simulink model "ThreePhaseVectorControl v2"  (R2020a)
settings: Solver=ode15s  StartTime=0.0  StopTime=2.5  MaxStep=1e-6  RelTol=1e-6
model workspace (MAT data in the model file):
  frequency = 1
values from neighbouring files (symbols this model uses):
  Buffer = 500    [PLLFYP.m]
  Ki_PLL = 0.005    [PLLFYP.m]
  Kp_PLL = 0.05    [PLLFYP.m]
  Kp_VSC = 500    [PLLFYP.m]
  Lf = 0.005    [PLLFYP.m]
  Lg = XR*Rg/(100*pi)    [PLLFYP.m]
  MPM_Ts = 1/5000    (= 0.0002)    [PLLFYP.m]
  Rf = 0.1    [PLLFYP.m]
  Rg = sqrt((1/(1+XR^2))*((500^2)/(Pn*SCR))^2)    [PLLFYP.m]
  Vdc = 2000    [PLLFYP.m]
  wL = 2*pi*50*Lf    (= 1.57079632679)    [PLLFYP.m]
  wn = 3000    [PLLFYP.m]
  zeta = 0.707    [PLLFYP.m]
undefined symbols (not defined in the file or in its folder): Ki_PQ, Kp_PQ, mpm_wc, plecs, Q, Q_KF, R, wb, wc, wc1, wc2
libraries: powerlib_meascontrol x57, powerlib x25, simulink x4, eeStairGenerator x4, powerlib_extras x2, cstblocks x2
(part 4 of 4)

== matlab function ThreePhaseVectorControl v2/Vector Current Controller + PWM/CF/MATLAB Function1 ==
  settings: updateMethod=DISCRETE
  data: G1 output; ROCOF input; clk input; G2 output
function [G1, G2]  = fcn(ROCOF, clk)

persistent time; persistent trig; persistent prev_G;   

if isempty(time)        % Initialize variables
    time = 0;
end
if isempty(trig)
    trig = 0;
end
if isempty(prev_G)
    prev_G = 0;
end

threshold = 2300;       % Set threshold to categorize dynamic/steady state

if (ROCOF < threshold)  % Steady state
    G1 = 0;
else 
    G1 = 1;             % dynamic
end

if (prev_G > G1)&&(trig == 0)       % Condition for switching from dynamic to steady state
    time = clk;
    G1 = 1;
    trig = 1;
elseif (prev_G > G1)&&(clk < time + 0.1)&&(trig == 1)   % Wait 0.1s before switching
    G1 = 1;
elseif (prev_G > G1)&&(clk == time + 0.1)&&(trig == 1)  % Switch
    G1 = 0;
    trig = 0;
elseif (prev_G == G1)&&(trig == 1)      % Start clock again if another dynamic event occurs
    time = clk;
end

G2 = 1 - G1;
prev_G = G1;

end

== matlab function ThreePhaseVectorControl v2/Vector Current Controller + PWM/CF/MATLAB Function2 ==
  data: G1 output; ROCOF input; G2 output
function [G1, G2] = fcn(ROCOF)

min_threshold = 1800;
max_threshold = 3500;

if (ROCOF < min_threshold)  % Steady state
    G1 = 0;
elseif (min_threshold <= ROCOF)&&(ROCOF < max_threshold)
    G1 = (ROCOF - min_threshold)/(max_threshold - min_threshold);
else 
    G1 = 1;
end

G2 = 1 - G1; % MPM weight

end

== matlab function ThreePhaseVectorControl v2/Vector Current Controller + PWM/KF_PLL/Kalman Filter-based PLL/Kalman Filter/KF_Vb ==
  data: Vb input; Vbk_S90 output; R input; Q input; w_k input; w_fk input
function Vbk_S90   = fcn(Vb, R, Q, w_k, w_fk)
 
persistent Phat;
persistent xhat;
 
if isempty(Phat)
      Phat = eye(6);
end
if isempty(xhat)
      xhat = zeros(6);
end

 
Ts = 10e-6;
 
a = sin(w_k*Ts)*sin(w_fk*Ts);
b = cos(w_k*Ts)*cos(w_fk*Ts);
c = sin(w_k*Ts)*cos(w_fk*Ts);
d = cos(w_k*Ts)*sin(w_fk*Ts);
e = sin(w_k*Ts);
f = cos(w_k*Ts);
phi_k = [b a d c 0 0; -a b -c -d 0 0; -d c b -a 0 0; -c d a b 0 0; 0 0 0 0 f e; 0 0 0 0 -e f];
F_k = [1 0 0 0 1 0];
 
% Time update
xhat_next = phi_k * xhat;
Phat_next = phi_k * Phat * phi_k' + Q;

% Kalman gain
K_k = 0.005*Phat_next * F_k' * inv(F_k*Phat_next*F_k' + R);

% Measurement update
xhat = xhat_next + K_k*(Vb - F_k*xhat_next);
Phat = Phat_next - K_k*F_k*Phat_next;

Vbk_S90 = xhat(6);

%K_k = phi_k * Phat * F_k' * (F_k*Phat*F_k' + R)^(-1);       % Compute Kalman gain
%xhat_next = phi_k * xhat + K_k*(Vb - F_k * xhat);           % Next state
%Phat_next = phi_k*Phat*phi_k' - K_k*F_k*Phat*phi_k' + ones(6)*Q;    % Predict state covariance
 
%Vbk_S90 = xhat_next(6);
 
%Phat = Phat_next;
%xhat = xhat_next;
 
end

== matlab function ThreePhaseVectorControl v2/Vector Current Controller + PWM/KF_PLL/Kalman Filter-based PLL/Kalman Filter/KF_Vc ==
  data: Vck_S90 output; Vc input; R input; Q input; w_k input; w_fk input
function Vck_S90  = fcn(Vc, R, Q, w_k, w_fk)
 
persistent Phat;
persistent xhat;
 
if isempty(Phat)
        Phat = eye(6);
end
if isempty(xhat)
        xhat = zeros(6);
end

Ts = 10e-6;
 
a = sin(w_k*Ts)*sin(w_fk*Ts);
b = cos(w_k*Ts)*cos(w_fk*Ts);
c = sin(w_k*Ts)*cos(w_fk*Ts);
d = cos(w_k*Ts)*sin(w_fk*Ts);
e = sin(w_k*Ts);
f = cos(w_k*Ts);
phi_k = [b a d c 0 0; -a b -c -d 0 0; -d c b -a 0 0; -c d a b 0 0; 0 0 0 0 f e; 0 0 0 0 -e f];
F_k = [1 0 0 0 1 0];

% Time update
xhat_next = phi_k * xhat;
Phat_next = phi_k * Phat * phi_k' + Q;

% Kalman gain
K_k = 0.005*Phat_next * F_k' * inv(F_k*Phat_next*F_k' + R);

% Measurement update
xhat = xhat_next + K_k*(Vc - F_k*xhat_next);
Phat = Phat_next - K_k*F_k*Phat_next;

Vck_S90 = xhat(6);

%K_k = phi_k * Phat * F_k' * (F_k*Phat*F_k' + R)^(-1);       % Compute Kalman gain
%xhat_next = phi_k * xhat + K_k*(Vc - F_k * xhat);           % Next state
%Phat_next = phi_k*Phat*phi_k' - K_k*F_k*Phat*phi_k' + ones(6)*Q;    % Predict state covariance
 
%Vck_S90 = xhat_next(6);
 
%x1k = xhat_next(1);                 % Flicker disturbance at n=1 freq
%x2k = xhat_next(2);                 % Flicker disturbance at n=2 freq
%x3k = xhat_next(3);                 % Flicker disturbance at n=3 freq
%x4k = xhat_next(4);                 % Flicker disturbance at n=4 freq
 
%Phat = Phat_next;
%xhat = xhat_next;
 
end

== matlab function ThreePhaseVectorControl v2/Vector Current Controller + PWM/FFT_PLL/FFT PLL ==
  data: data input; f output; T input
function f = fcn(data, T)

%data = detrend(data,0);

f = 0;

Fs = 1/T;
N = length(data);

NFFT = 2^nextpow2(N); % Next power of 2 from length of y
Y = fft(data,NFFT)/N;
fz = Fs/2*linspace(0,1,NFFT/2+1);
Y_new = 2*abs(Y(1:NFFT/2+1));

[temp, i] = max(Y_new);
f = fz(i);





% NFFT = 2 ^ nextpow2(N);             % Compute FFT length
% Y = fft(data, NFFT);   % Compute FFT of signal
% Y = Y(1:NFFT/2);                    % Take one side of FFT plot
% Y_abs = 1/NFFT*abs(Y);              % Calculate magnitude and normalize the spectrum
% f_fft = (0:NFFT/2-1)*Fs/NFFT;       % Scale the frequency axis
% 
% [m, i] = max(Y_abs);    % Find peak frequency
% % % 
% f = f_fft(i);           % Output the corresponding frequency of the peak


% f = 0;
% 
% T = 10e-6;
% Fs = 1/T;
% L = size(data,1);
% 
% Y = fft(data);
% Y = abs(Y/L);
% X = Y(1:L/2+1);
% X(2:end-1) = 2*X(2:end-1);
% fr = Fs*(0:(L/2))/L;
% 
% %plot(fr, X)          % Plot frequency
% 
% [m, i] = max(X);     % Find peak frequency
% 
% f = fr(i);           % Output the corresponding frequency of the peak

== matlab function ThreePhaseVectorControl v2/Vector Current Controller + PWM/KF_PLL/KF//GAM/Kalman Filter/KF_Va ==
  data: y_k input; v_fk output; R input; Q input; w_k input; V_fk_S90 output
function [v_fk, V_fk_S90] = fcn(y_k, R, Q, w_k)
 
persistent P_k;
persistent xhat_k;

% Initialize xhat and Phat
    if isempty(P_k)
        P_k = eye(2, 2); %eye(2);
    end
    if isempty(xhat_k)
        xhat_k = zeros(2, 1);
    end
    
% Variables for KF
    Ts = 10e-6;       
    phi_k = [cos(w_k*Ts) sin(w_k*Ts); -sin(w_k*Ts) cos(w_k*Ts)]; 
    F_k = [1 0];


K = phi_k * P_k * F_k' / (F_k * P_k * F_k' + R);        %K_gain * Phat_next * F_k' /(F_k*Phat_next*F_k' + R);    
xhat_k1 = phi_k * xhat_k + K * (y_k - F_k * xhat_k);
P_k1 = phi_k * P_k * phi_k' - K * F_k * P_k * phi_k' + Q;

xhat_k = xhat_k1;
P_k = P_k1;

% Output
v_fk = xhat_k1(1);
V_fk_S90 = xhat_k1(2);


 
end

== matlab function ThreePhaseVectorControl v2/Vector Current Controller + PWM/KF_PLL/Kalman Filter-based PLL/Kalman Filter/KF_Va ==
  data: Va input; Vak_S90 output; R input; Q input; w_k input; w_fk input
function Vak_S90    = fcn(Va, R, Q, w_k, w_fk)
 
persistent Phat;
persistent xhat;

if isempty(Phat)
    Phat = eye(6);
end
if isempty(xhat)
    xhat = zeros(6);
end


Ts = 10e-6;
 
a = sin(w_k*Ts)*sin(w_fk*Ts);
b = cos(w_k*Ts)*cos(w_fk*Ts);
c = sin(w_k*Ts)*cos(w_fk*Ts);
d = cos(w_k*Ts)*sin(w_fk*Ts);
e = sin(w_k*Ts);
f = cos(w_k*Ts);
phi_k = [b a d c 0 0; -a b -c -d 0 0; -d c b -a 0 0; -c d a b 0 0; 0 0 0 0 f e; 0 0 0 0 -e f];
F_k = [1 0 0 0 1 0];
 
% Time update
xhat_next = phi_k * xhat;
Phat_next = phi_k * Phat * phi_k' + Q;

% Kalman gain
K_k = 0.005*Phat_next * F_k' * inv(F_k*Phat_next*F_k' + R);

% Measurement update
xhat = xhat_next + K_k*(Va - F_k*xhat_next);
Phat = Phat_next - K_k*F_k*Phat_next;

Vak_S90 = xhat(6);



%K_k = phi_k * Phat * F_k' * (F_k*Phat*F_k' + R)^(-1);       % Compute Kalman gain
%xhat_next = phi_k * xhat + K_k*(Va - F_k * xhat);           % Next state
%Phat_next = phi_k*Phat*phi_k' - K_k*F_k*Phat*phi_k' + ones(6)*Q;    % Predict state covariance

%Vak_S90 = xhat_next(6);

%Phat = Phat_next;
%xhat = xhat_next;
 
end

== matlab function ThreePhaseVectorControl v2/Vector Current Controller + PWM/CF based on i_d/CF_func ==
  data: i_d input; MPM input; SRF input; CF_freq output; FFT_freq input
function CF_freq = fcn(i_d, MPM, SRF, FFT_freq)

g1 = 0;
g2 = 0;

if (i_d < 10)
    g1 = 1;
    g2 = 0;
elseif (10 <= i_d)&&(i_d < 15)
    g1 = 0;
    g2 = 0;
elseif (15 <= i_d)&&(i_d < 20)
    g1 = 0;
    g2 = (i_d-15)/5;
else
    g1 = 0;
    g2 = 1;
end

f = g1 * SRF + (1-g1-g2) * MPM + g2 * FFT_freq;

CF_freq = f;

== matlab function ThreePhaseVectorControl v2/Vector Current Controller + PWM/MPM CF/MPM/MPM 0.5 cycle ==
  data: x input; L input; timestep input; freq_guess input; outputfreq output; cycle5_freq input
function outputfreq = Our_MPM_QR_pca(x,L,timestep,freq_guess, cycle5_freq)

%     Applies the Total Forward Backward Matrix Pencil Method to resolve the
%     synchrophasor of an input signal
%     Author: Lakshan Bernard, Sunny Goondram

% Inputs
% x:          one window of the timeseries
% L:          pencil parameter
% timestep:   time between sample points
% freq_guess: which phasors to report. NB: the method calculates all phasors
%             but the this just tells the algorithm to output phasor closest
%             to freq_guess
%             
% Outputs
% outputphasor:   a complex number representing the phasor relative to start
%                 of the window.
% outputfreq:     the frequency of the phasor. Note this is different to
%                 freq_guess
% eigS, residues: these contain all the frequency and phasor data

x = reshape(x, [], 1); %reshape data into column vector
N = length(x);
sampleoffset = (ceil(N/2)+1);
xold = x;

persistent f0;
if isempty(f0)
    f0 = freq_guess;
end

% Hyperparameters
DYNAMIC = 0;
if(DYNAMIC)
    epsilon=0.125;
    sys_order=floor((0.22/(50*timestep)));
else
    epsilon= 0.725;  %0.0050;
    sys_order=floor((N-sampleoffset)*1);
end

%% Filtering
    L1 = ceil(N/2);
    Y = hankel(x(1:N-L1), x(N-L1:N)); diagIdx = (N:-1:1)-L1;
    
    Y_mean = mean(Y,1);
    n = size(Y,1);
    matrix_mean = repmat(Y_mean,n,1); %creates a matrix with similar rows 
    centered_data = Y- matrix_mean;% centering the data by subtracting the mean
    M = ((centered_data')*centered_data)/(n-1);
    [V,D] = eig(M); %V are eigenvectors and D represents the eigenvalues 

    %sorting the eigen values in descending order
    lx = size(Y,2);
    eval = zeros(1,lx);
    eval = complex(eval, zeros(size(eval), class(eval)) );                      % Additional code added in
    for k = 1:lx
        eval(1,k) = D(k,k);
    end 
    [eval_sorted,I] = sort(eval,'descend');
    
    S = cumsum(abs(eval_sorted));
    limit = find((S/S(end))>0.9999999,1);
    if isempty(limit)                                                           % Additional code added in
        limit = 1;
    end
    limit = limit(1);
    evec_sorted = zeros(lx,limit);
    evec_sorted = complex(evec_sorted, zeros(size(evec_sorted), class(evec_sorted)) );    % Additional code added in
    for m =1:limit
        evec_sorted(:,m) = V(:,I(m));
    end
        
    %reconstruction
    princ_compon_limit = centered_data*evec_sorted;
    reconstructed = princ_compon_limit *(evec_sorted');
    reconstructed = reconstructed + matrix_mean;
    C = reconstructed;
 
    x1 = zeros(1,N);
    x1 = complex(x1, zeros(size(x1), class(x1)) );                              % Additional code added in
    for i=1:length(diagIdx) %averaging antidiagonals
        x1(i) = mean(diag(fliplr(C),diagIdx(i)));
    end    
    C = hankel(x1(1:N-L1), x1(N-L1:N)); 

    
%% Solving GEP

%perform the Column permutated QR decomposition for finding eigenvalues
%find the QR decomp for the all data matrix
[Q,R,E]=qr(C);

%rank estimation
order=0;

for i=1:length(diag(R))
    if abs(R(i,i))>=epsilon*abs(R(1,1))
        order=order+1;
    end
end

% Use permutation matrix to modify the Triangular R matrix
S=R*((E).');
% Create a new truncated pencil using the new matrix 
T1=S(1:order,1:L);
T2=S(1:order,2:L+1);
%modify the new pencil with diagonal of R matrix
Dinv=inv(diag(diag(R(1:order,1:order))));
T1dash=Dinv*T1;
T2dash=Dinv*T2;
%use the new pencil to find the eigenvalues
eigsS=eig(pinv(T2dash)*T1dash);
%remove the 0 eigenvalues;

eigsS(abs(eigsS)<10^-8)=[];
eigsS((abs(eigsS)<0.9)|(abs(eigsS)>1.1))=0;
order=length(eigsS);

%% Solving Complex Amplitudes
%form the linear system to solve for the complex amplitudes
ans_vec=xold(1+sampleoffset:sys_order+sampleoffset); %build answer vector (NB, this data hasnt been filtered :/)
coef_mat=zeros(sys_order,order);
coef_mat = complex(coef_mat, zeros(size(coef_mat), class(coef_mat)) );         % Additional code added in
for i=1:sys_order %build coefficient matrix
    for j=1:order
        coef_mat(i,j)=eigsS(j)^(i-1);
    end
end
residues=pinv(coef_mat)*ans_vec; %find the complex amplitudes


%% Estimating Frequency
freq = angle(eigsS)/(2*pi*timestep);
estfreq=freq_guess; %to report fundamental phasor replace with 50..
outputfreq_temp = mean(freq( (freq>0.2*estfreq)&(freq<2.0*estfreq) )); %mean(freq( (freq>0.85*estfreq)&(freq<1.15*estfreq) ));

if (outputfreq_temp < 100)&&(outputfreq_temp > 0)
    f0 = outputfreq_temp;
else
    outputfreq_temp = cycle5_freq;
end
 
 outputfreq = outputfreq_temp;

%% Reconstructing Phasor
%outputphasor = 2*sum(residues( (freq>0.85*freq_guess)&(freq<1.15*freq_guess) ));

== matlab function ThreePhaseVectorControl v2/Vector Current Controller + PWM/MPM CF/MPM/MPM 5 cycle ==
  data: x input; L input; timestep input; freq_guess input; outputfreq output
function outputfreq = Our_MPM_QR_pca(x,L,timestep,freq_guess)

%     Applies the Total Forward Backward Matrix Pencil Method to resolve the
%     synchrophasor of an input signal
%     Author: Lakshan Bernard, Sunny Goondram

% Inputs
% x:          one window of the timeseries
% L:          pencil parameter
% timestep:   time between sample points
% freq_guess: which phasors to report. NB: the method calculates all phasors
%             but the this just tells the algorithm to output phasor closest
%             to freq_guess
%             
% Outputs
% outputphasor:   a complex number representing the phasor relative to start
%                 of the window.
% outputfreq:     the frequency of the phasor. Note this is different to
%                 freq_guess
% eigS, residues: these contain all the frequency and phasor data

x = reshape(x, [], 1); %reshape data into column vector
N = length(x);
sampleoffset = (ceil(N/2)+1);
xold = x;

% Hyperparameters
DYNAMIC = 0;
if(DYNAMIC)
    epsilon=0.125;
    sys_order=floor((0.22/(50*timestep)));
else
    epsilon=0.725; %0.0050;
    sys_order=floor((N-sampleoffset)*1);
end

%% Filtering
    L1 = ceil(N/2);
    Y = hankel(x(1:N-L1), x(N-L1:N)); diagIdx = (N:-1:1)-L1;
    
    Y_mean = mean(Y,1);
    n = size(Y,1);
    matrix_mean = repmat(Y_mean,n,1); %creates a matrix with similar rows 
    centered_data = Y- matrix_mean;% centering the data by subtracting the mean
    M = ((centered_data')*centered_data)/(n-1);
    [V,D] = eig(M); %V are eigenvectors and D represents the eigenvalues 

    %sorting the eigen values in descending order
    lx = size(Y,2);
    eval = zeros(1,lx);
    eval = complex(eval, zeros(size(eval), class(eval)) );                      % Additional code added in
    for k = 1:lx
        eval(1,k) = D(k,k);
    end 
    [eval_sorted,I] = sort(eval,'descend');
    
    S = cumsum(abs(eval_sorted));
    limit = find((S/S(end))>0.9999999,1);
    if isempty(limit)                                                           % Additional code added in
        limit = 1;
    end
    limit = limit(1);
    evec_sorted = zeros(lx,limit);
    evec_sorted = complex(evec_sorted, zeros(size(evec_sorted), class(evec_sorted)) );    % Additional code added in
    for m =1:limit
        evec_sorted(:,m) = V(:,I(m));
    end
        
    %reconstruction
    princ_compon_limit = centered_data*evec_sorted;
    reconstructed = princ_compon_limit *(evec_sorted');
    reconstructed = reconstructed + matrix_mean;
    C = reconstructed;
 
    x1 = zeros(1,N);
    x1 = complex(x1, zeros(size(x1), class(x1)) );                              % Additional code added in
    for i=1:length(diagIdx) %averaging antidiagonals
        x1(i) = mean(diag(fliplr(C),diagIdx(i)));
    end    
    C = hankel(x1(1:N-L1), x1(N-L1:N)); 

    
%% Solving GEP

%perform the Column permutated QR decomposition for finding eigenvalues
%find the QR decomp for the all data matrix
[Q,R,E]=qr(C);

%rank estimation
order=0;

for i=1:length(diag(R))
    if abs(R(i,i))>=epsilon*abs(R(1,1))
        order=order+1;
    end
end

% Use permutation matrix to modify the Triangular R matrix
S=R*((E).');
% Create a new truncated pencil using the new matrix 
T1=S(1:order,1:L);
T2=S(1:order,2:L+1);
%modify the new pencil with diagonal of R matrix
Dinv=inv(diag(diag(R(1:order,1:order))));
T1dash=Dinv*T1;
T2dash=Dinv*T2;
%use the new pencil to find the eigenvalues
eigsS=eig(pinv(T2dash)*T1dash);
%remove the 0 eigenvalues;

eigsS(abs(eigsS)<10^-8)=[];
eigsS((abs(eigsS)<0.9)|(abs(eigsS)>1.1))=0;
order=length(eigsS);

%% Solving Complex Amplitudes
%form the linear system to solve for the complex amplitudes
ans_vec=xold(1+sampleoffset:sys_order+sampleoffset); %build answer vector (NB, this data hasnt been filtered :/)
coef_mat=zeros(sys_order,order);
coef_mat = complex(coef_mat, zeros(size(coef_mat), class(coef_mat)) );         % Additional code added in
for i=1:sys_order %build coefficient matrix
    for j=1:order
        coef_mat(i,j)=eigsS(j)^(i-1);
    end
end
residues=pinv(coef_mat)*ans_vec; %find the complex amplitudes


%% Estimating Frequency
freq = angle(eigsS)/(2*pi*timestep);
estfreq=freq_guess; %to report fundamental phasor replace with 50..
outputfreq = mean(freq( (freq>0.85*estfreq)&(freq<1.15*estfreq) ));

%% Reconstructing Phasor
%outputphasor = 2*sum(residues( (freq>0.85*freq_guess)&(freq<1.15*freq_guess) ));

== matlab function ThreePhaseVectorControl v2/Vector Current Controller + PWM/KF_PLL/KF//GAM/Kalman Filter/KF_Va1 ==
  data: Va input; Vb input; Vc input; Vak output; R input; Q input; w_k input; Vbk output; Vck output; K_gain input
function [Vak, Vbk, Vck] = fcn(Va, Vb, Vc, R, Q, w_k, K_gain)
 
persistent Phat_a; persistent Phat_b; persistent Phat_c;
persistent xhat_a; persistent xhat_b; persistent xhat_c;

% Initialize xhat and Phat
    if isempty(Phat_a)
        Phat_a = eye(2);
    end
    if isempty(Phat_b)
        Phat_b = eye(2);
    end
    if isempty(Phat_c)
        Phat_c = eye(2);
    end
    if isempty(xhat_a)
        xhat_a = zeros(2, 1);
    end
    if isempty(xhat_b)
        xhat_b = zeros(2, 1);
    end
    if isempty(xhat_c)
        xhat_c = zeros(2, 1);
    end
    
% Initialize w_k to 2*pi*50 for 40us
%     if isempty(w_k)
%         w_k = 2*pi*50;
%     end

% Variables & matrices for KF
    Ts = 10e-6;        % time period = 10 us
    phi_k = [cos(w_k*Ts) sin(w_k*Ts); -sin(w_k*Ts) cos(w_k*Ts)];  %phi_k = [1 0; 0 1];
    F_k = [1 0];

%%%%%%%%%%%%%%%%%%%%% KF for Va %%%%%%%%%%%%%%%%%%%%%
% Time update
xhat_a_next = phi_k * xhat_a;
Phat_a_next = phi_k * Phat_a * phi_k' + Q;

% Kalman gain
K_a = K_gain*Phat_a_next * F_k' /(F_k*Phat_a_next*F_k' + R);

% Measurement update
xhat_a = xhat_a_next + K_a*(Va - F_k*xhat_a_next);
Phat_a = Phat_a_next - K_a*F_k*Phat_a_next;


%%%%%%%%%%%%%%%%%%%%% KF for Vb %%%%%%%%%%%%%%%%%%%%%
% Time update
xhat_b_next = phi_k * xhat_b;
Phat_b_next = phi_k * Phat_b * phi_k' + Q;

% Kalman gain
K_b = K_gain*Phat_b_next * F_k' /(F_k*Phat_b_next*F_k' + R);

% Measurement update
xhat_b = xhat_b_next + K_b*(Vb - F_k*xhat_b_next);
Phat_b = Phat_b_next - K_b*F_k*Phat_b_next;

%%%%%%%%%%%%%%%%%%%%% KF for Vc %%%%%%%%%%%%%%%%%%%%%
% Time update
xhat_c_next = phi_k * xhat_c;
Phat_c_next = phi_k * Phat_c * phi_k' + Q;

% Kalman gain
K_c = K_gain*Phat_c_next * F_k' /(F_k*Phat_c_next*F_k' + R);

% Measurement update
xhat_c = xhat_c_next + K_c*(Vc - F_k*xhat_c_next);
Phat_c = Phat_c_next - K_c*F_k*Phat_c_next;


% Output
Vak = xhat_a(1);
Vbk = xhat_b(1);
Vck = xhat_c(1);

 
end
